simulink model "simulate"  (R2017b)
settings: Solver=FixedStepAuto  StartTime=0.0  StopTime=70  FixedStep=0.01  RelTol=1e-3
PreLoadFcn:
  | bus_definitions
settings Model: Creator=petter  LastModifiedBy=petter

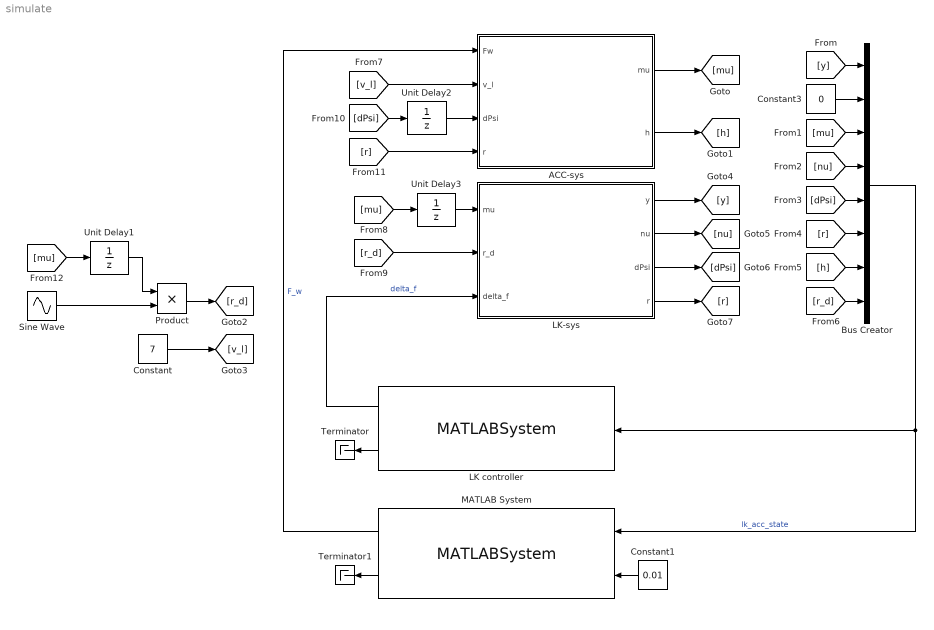
== system simulate ==
  ACC-sys : Subsystem
  Bus Creator : BusCreator  Inputs=8  OutDataTypeStr=Bus: LKACCBus
      settings: InheritFromInputs=off
  Constant : Constant  Value=7
  Constant1 : Constant  Value=0.01
  Constant3 : Constant  Value=0
  LK controller : MATLABSystem  System=lk_pcis_controller  H_x=diag([1 0 0.25 0])  f_x=[0;0;0;0]  H_u=4  f_u=0  M=1800  lf=1.2  lr=1.650  Caf=140000  Car=120000  Iz=3270.0  sol_opts=struct( 'DataType', 'double', 'MaxIter', 200, 'FeasibilityTol', 1e-6, 'IntegrityChecks', true )  SimulateUsing=Code generation
      mask Type: lk_pcis_controller
      mask Display:
      | disp('lk_pcis_controller');
      | port_label('input',1,'lk_acc_state');
      | port_label('output',1,'delta_f');
      | port_label('output',2,'control_info');
  LK-sys : Subsystem
  MATLAB System : MATLABSystem  System=acc_pcis_controller  M=1800  f0bar=74.63  f1bar=40.59  vl=7  v_des=8  M_p=1  M_d=0  M_i=0  K_i=0  sol_opts=struct( 'DataType', 'double', 'MaxIter', 200, 'FeasibilityTol', 1e-6, 'IntegrityChecks', true )  SimulateUsing=Code generation
      mask Type: acc_pcis_controller
      mask Display:
      | disp('acc_pcis_controller');
      | port_label('input',1,'lk_acc_state');
      | port_label('input',2,'dt');
      | port_label('output',1,'F_w');
      | port_label('output',2,'control_info');
  Product : Product
  Sine Wave : Sin  Amplitude=0.03  Frequency=pi/10  SampleTime=0
  Terminator : Terminator
  Terminator1 : Terminator
  Unit Delay1 : UnitDelay  SampleTime=-1
  Unit Delay2 : UnitDelay  SampleTime=-1
  Unit Delay3 : UnitDelay  SampleTime=-1
  wires:
  LK controller/1 -> LK-sys/3(delta_f)  "delta_f"
  Bus Creator/1 -> LK controller/1, MATLAB System/1  "lk_acc_state"
  ACC-sys/1(mu) -> [mu]
  ACC-sys/2(h) -> [h]
  Constant/1 -> [v_l]
  LK-sys/1(y) -> [y]
  LK-sys/2(nu) -> [nu]
  LK-sys/3(dPsi) -> [dPsi]
  LK-sys/4(r) -> [r]
  [y] -> Bus Creator/1
  [mu] -> Bus Creator/3
  [nu] -> Bus Creator/4
  [dPsi] -> Bus Creator/5
  [r] -> Bus Creator/6
  [h] -> Bus Creator/7
  [r_d] -> Bus Creator/8
  [v_l] -> ACC-sys/2(v_l)
  [mu] -> Unit Delay3/1
  Constant1/1 -> MATLAB System/2
  [dPsi] -> Unit Delay2/1
  [r] -> ACC-sys/4(r)
  MATLAB System/1 -> ACC-sys/1(Fw)  "F_w"
  Unit Delay2/1 -> ACC-sys/3(dPsi)
  Unit Delay3/1 -> LK-sys/1(mu)
  Constant3/1 -> Bus Creator/2
  LK controller/2 -> Terminator/1
  MATLAB System/2 -> Terminator1/1
  [r_d] -> LK-sys/2(r_d)
  [mu] -> Unit Delay1/1
  Product/1 -> [r_d]
  Sine Wave/1 -> Product/2
  Unit Delay1/1 -> Product/1

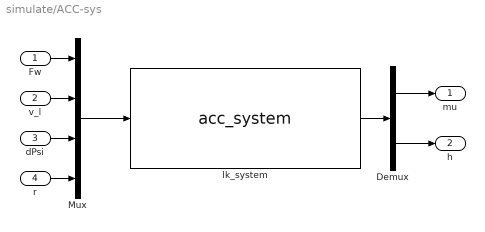
== system simulate/ACC-sys ==
  Fw : Inport
  v_l : Inport  Port=2
  dPsi : Inport  Port=3
  r : Inport  Port=4
  Demux : Demux  Outputs=2
  Mux : Mux
  lk_system : S-Function  FunctionName=acc_system  Parameters=[7;40]  SFunctionDeploymentMode=off  EnableBusSupport=off
  mu : Outport
  h : Outport  Port=2
  wires:
  Mux/1 -> lk_system/1
  Fw/1 -> Mux/1
  v_l/1 -> Mux/2
  lk_system/1 -> Demux/1
  Demux/1 -> mu/1
  Demux/2 -> h/1
  dPsi/1 -> Mux/3
  r/1 -> Mux/4

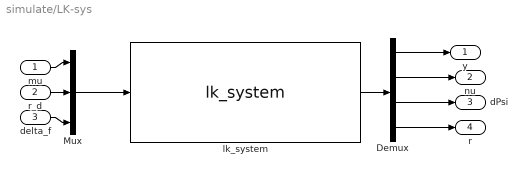
== system simulate/LK-sys ==
  mu : Inport
  r_d : Inport  Port=2
  delta_f : Inport  Port=3
  Demux : Demux
  Mux : Mux  Inputs=3
  lk_system : S-Function  FunctionName=lk_system  Parameters=[0;0;0;0]  SFunctionDeploymentMode=off  EnableBusSupport=off
  y : Outport
  nu : Outport  Port=2
  dPsi : Outport  Port=3
  r : Outport  Port=4
  wires:
  Mux/1 -> lk_system/1
  mu/1 -> Mux/1
  r_d/1 -> Mux/2
  delta_f/1 -> Mux/3
  lk_system/1 -> Demux/1
  Demux/1 -> y/1
  Demux/2 -> nu/1
  Demux/3 -> dPsi/1
  Demux/4 -> r/1
